simulink model "tarea2"  (R2021a)
settings: Solver=ode4  StartTime=0.0  StopTime=10.0  FixedStep=1e-3  RelTol=1e-3
libraries: simulink x1
settings Model: Creator=frand  LastModifiedBy=frand

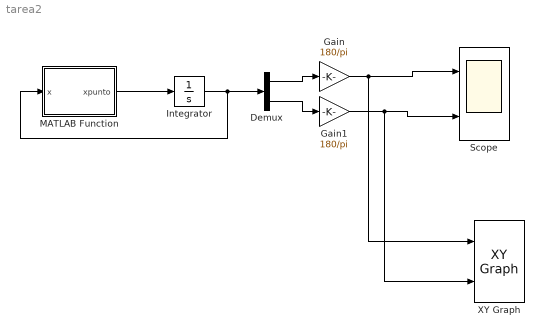
== system tarea2 ==
  Demux : Demux  Outputs=2
  Gain : Gain  Gain=180/pi
  Gain1 : Gain  Gain=180/pi
  Integrator : Integrator  InitialCondition=[-pi+180/pi;0]
  MATLAB Function : MATLAB Function  TreatAsAtomicUnit=on
  Scope : Scope  NumInputPorts=2
  XY Graph : simulink/Sinks/XY Graph  xmin=3200  xmax=3500  ymin=-40  ymax=80  st=-1
  wires:
  MATLAB Function/1(xpunto) -> Integrator/1
  Demux/2 -> Gain1/1
  Demux/1 -> Gain/1
  Integrator/1 -> Demux/1, MATLAB Function/1(x)
  Gain/1 -> XY Graph/1, Scope/1
  Gain1/1 -> XY Graph/2, Scope/2

== matlab function tarea2/MATLAB Function ==
  data: x input; xpunto output
function xpunto = f(x)
b = 0.5;
xpunto = [x(2);sin(x(1))-b*x(2)];
